simulink model "final_ekf_switch_test"  (R2024a)
settings: Solver=VariableStepAuto  StartTime=0.0  StopTime=10.0  RelTol=1e-3
undefined symbols (not defined in the file): DiscIntNeverNeededParam, g_val, Ki, Kx, m_val, r_pos
libraries: sharedTrackingLibrary x1
settings Model: Creator=yufon  LastModifiedBy=yufon

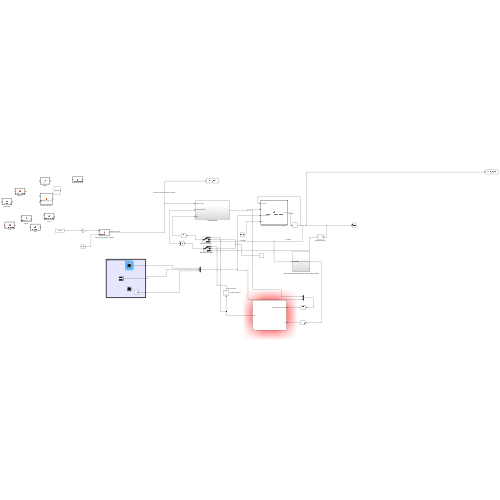
[thumbnail: Simulink's stored preview of the top-level diagram]
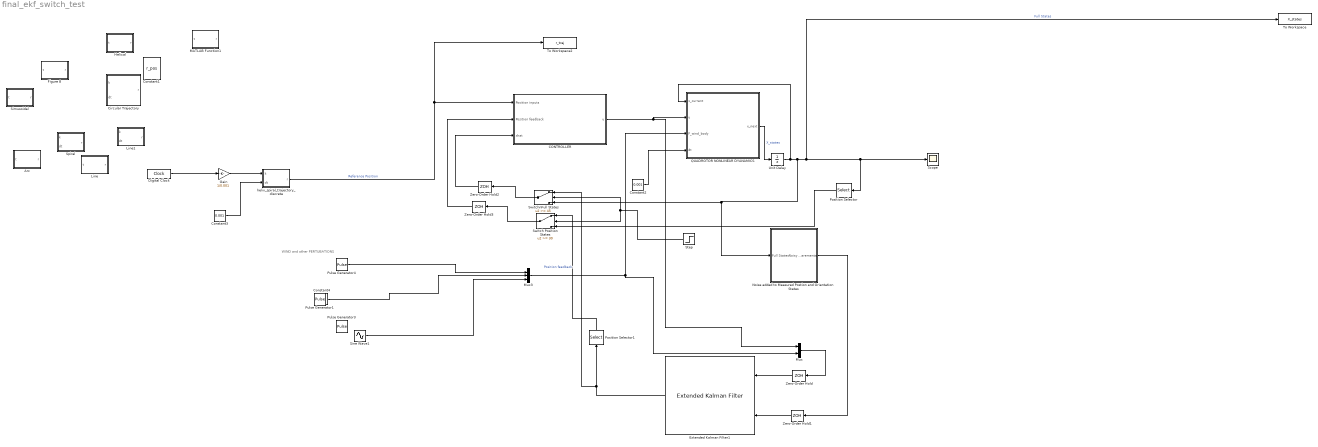
== system final_ekf_switch_test ==
  note: WIND and other PERTUBATIONS
  Arc : MATLAB Function  TreatAsAtomicUnit=on
  CONTROLLER : Subsystem
  Circular Trajectory : MATLAB Function  TreatAsAtomicUnit=on
  Constant1 : Constant  Value=r_pos  VectorParams1D=off
  Constant2 : Constant  Value=0.001
  Constant3 : Constant  Value=0.001
  Constant4 : Constant  Value=0
  Digital Clock : DigitalClock  SampleTime=0.01
  Extended Kalman Filter1 : sharedTrackingLibrary/Extended Kalman Filter  StateTransitionFcn=myStateTransitionFcn  HasStateTransitionJacobianFcn=off  HasAdditiveProcessNoise=Additive  ProcessNoise=Q  HasTimeVaryingProcessNoise=off  HasStateTransitionFcnExtraArgument=1  InitialState=EKF_x0  InitialStateCovariance=P0  MeasurementFcn1=myMeasurementFcn  HasMeasurementJacobianFcn1=off  HasMeasurementEnablePort1=off  HasAdditiveMeasurementNoise1=Additive  MeasurementNoise1=R  HasTimeVaryingMeasurementNoise1=off  HasMeasurementFcnExtraArgument1=0  HasMeasurementWrapping1=off  MeasurementFcn2=myMeasurementFcn  HasMeasurementJacobianFcn2=off  HasMeasurementEnablePort2=off  HasAdditiveMeasurementNoise2=Additive  MeasurementNoise2=1  HasTimeVaryingMeasurementNoise2=off  HasMeasurementFcnExtraArgument2=0  HasMeasurementWrapping2=off  MeasurementFcn3=myMeasurementFcn  HasMeasurementJacobianFcn3=off  HasMeasurementEnablePort3=off  HasAdditiveMeasurementNoise3=Additive  MeasurementNoise3=1  HasTimeVaryingMeasurementNoise3=off  HasMeasurementFcnExtraArgument3=0  HasMeasurementWrapping3=off  MeasurementFcn4=myMeasurementFcn  HasMeasurementJacobianFcn4=off  HasMeasurementEnablePort4=off  HasAdditiveMeasurementNoise4=Additive  MeasurementNoise4=1  HasTimeVaryingMeasurementNoise4=off  HasMeasurementFcnExtraArgument4=0  HasMeasurementWrapping4=off  MeasurementFcn5=myMeasurementFcn  HasMeasurementJacobianFcn5=off  HasMeasurementEnablePort5=off  HasAdditiveMeasurementNoise5=Additive  MeasurementNoise5=1  HasTimeVaryingMeasurementNoise5=off  HasMeasurementFcnExtraArgument5=0  HasMeasurementWrapping5=off  EnableMultirate=off  StateTransitionFcnSampleTime=1  MeasurementFcn1SampleTime=1  MeasurementFcn2SampleTime=1  MeasurementFcn3SampleTime=1  MeasurementFcn4SampleTime=1  MeasurementFcn5SampleTime=1  UseCurrentEstimator=on  OutputStateCovariance=off  DataType=double  SampleTime=0.001  NumberOfMeasurements=1
  Figure 8 : MATLAB Function  TreatAsAtomicUnit=on
  Gain : Gain  Gain=1/0.001
  Helical : MATLAB Function  TreatAsAtomicUnit=on
  Line : MATLAB Function  TreatAsAtomicUnit=on
  Line1 : MATLAB Function  TreatAsAtomicUnit=on
  MATLAB Function1 : MATLAB Function  TreatAsAtomicUnit=on
  Mux : Mux  Inputs=2
  Mux3 : Mux  Inputs=3
  Noise added to Measured Postion and Orientation States : Subsystem
  Position Selector : Selector  InputPortWidth=12  IndexOptions=Index vector (dialog)  Indices=[1 2 3]  OutputSizes=1
  Position Selector1 : Selector  InputPortWidth=12  IndexOptions=Index vector (dialog)  Indices=[1 2 3]  OutputSizes=1
  Pulse Generator1 : DiscretePulseGenerator  Amplitude=10  Period=10  PulseWidth=5  PhaseDelay=20  SampleTime=10
  Pulse Generator3 : DiscretePulseGenerator  PulseType=Time based  Amplitude=3  Period=5  PhaseDelay=100
  Pulse Generator4 : DiscretePulseGenerator  PulseType=Time based  Amplitude=3  Period=10  PulseWidth=5  PhaseDelay=50
  QUADROTOR NONLINEAR DYANAMICS : MATLAB Function  TreatAsAtomicUnit=on
  Scope : Scope
  Simusoidal : MATLAB Function  TreatAsAtomicUnit=on
  Sine Wave1 : Sin  Amplitude=5  Frequency=0.5  SampleTime=0
  Spiral : MATLAB Function  TreatAsAtomicUnit=on
  Step : Step  Time=45  After=30  SampleTime=0.001
  Switch Position States : Switch  Threshold=30  SaturateOnIntegerOverflow=off  InputSameDT=off
  SwitchnFull States : Switch  Threshold=45  SaturateOnIntegerOverflow=off  InputSameDT=off
  To Workspace : ToWorkspace  VariableName=X_states  SampleTime=-1
  To Workspace2 : ToWorkspace  VariableName=r_traj  SaveFormat=Timeseries  SampleTime=-1
  Unit Delay : UnitDelay  SampleTime=0.001  HasFrameUpgradeWarning=on
  Zero-Order Hold{,1..3} (4 alike) : ZeroOrderHold  SampleTime=0.001
  helix_spiral_trajectory_discrete : MATLAB Function  TreatAsAtomicUnit=on
  wires:
  Unit Delay/1 -> SwitchnFull States/3, Noise added to Measured Postion and Orientation States/1(Full States), Position Selector/1, Scope/1, To Workspace/1, QUADROTOR NONLINEAR DYANAMICS/1(x_current)  "Full States"
  SwitchnFull States/1 -> Zero-Order Hold2/1
  Extended Kalman Filter1/1 -> SwitchnFull States/1, Position Selector1/1
  helix_spiral_trajectory_discrete/1(r) -> To Workspace2/1, CONTROLLER/1(Position inputs)  "Reference Position"
  Constant3/1 -> helix_spiral_trajectory_discrete/2(dt)
  Zero-Order Hold3/1 -> CONTROLLER/2(Position feedback)
  Constant2/1 -> QUADROTOR NONLINEAR DYANAMICS/4(dt)
  Digital Clock/1 -> Gain/1
  Mux3/1 -> Mux/2, QUADROTOR NONLINEAR DYANAMICS/3(F_wind_body)
  Zero-Order Hold1/1 -> Extended Kalman Filter1/2
  Zero-Order Hold2/1 -> CONTROLLER/3(xhat)
  Mux/1 -> Zero-Order Hold/1
  Step/1 -> SwitchnFull States/2, Switch Position States/2
  Gain/1 -> helix_spiral_trajectory_discrete/1(k)
  Sine Wave1/1 -> Mux3/3
  CONTROLLER/1(u) -> Mux/1, QUADROTOR NONLINEAR DYANAMICS/2(u)
  Zero-Order Hold/1 -> Extended Kalman Filter1/1
  Constant4/1 -> Mux3/2
  Pulse Generator4/1 -> Mux3/1
  Position Selector/1 -> Switch Position States/3
  Position Selector1/1 -> Switch Position States/1  "Position feedback"
  Switch Position States/1 -> Zero-Order Hold3/1
  QUADROTOR NONLINEAR DYANAMICS/1(x_next) -> Unit Delay/1  "X_states"
  Noise added to Measured Postion and Orientation States/1(Noisy Position and Orientation Mesuarements) -> Zero-Order Hold1/1

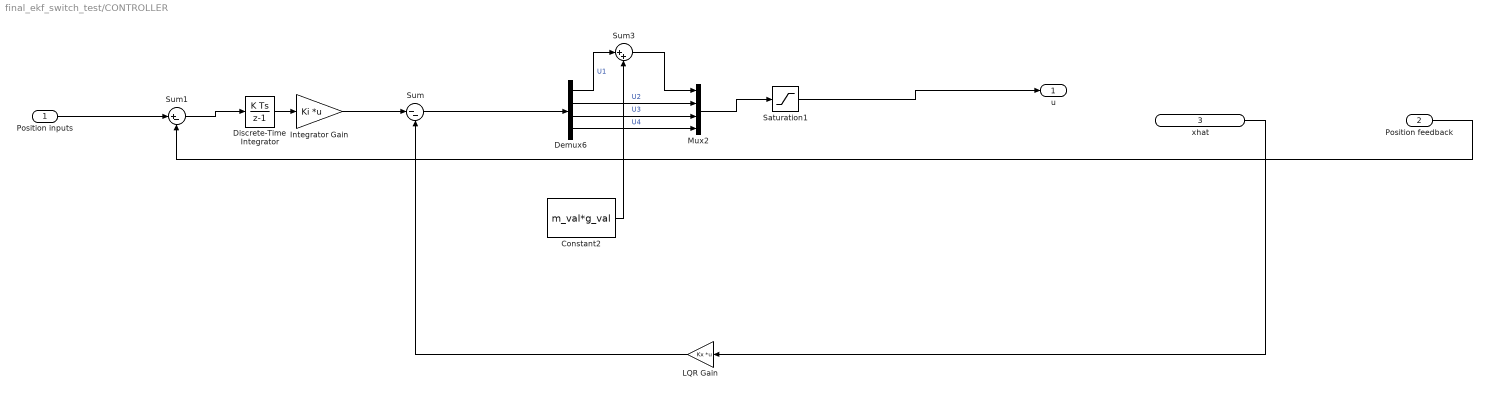
== system final_ekf_switch_test/CONTROLLER ==
  Position inputs : Inport
  Position feedback : Inport  Port=2
  xhat : Inport  Port=3
  Constant2 : Constant  Value=m_val*g_val
  Demux6 : Demux
  Discrete-Time Integrator : DiscreteIntegrator  SampleTime=0.001  ICPrevOutput=DiscIntNeverNeededParam  ICPrevScaledInput=DiscIntNeverNeededParam
  Integrator Gain : Gain  Gain=Ki  Multiplication=Matrix(K*u)
  LQR Gain : Gain  Gain=Kx  Multiplication=Matrix(K*u)
  Mux2 : Mux
  Saturation1 : Saturate  UpperLimit=[40; 0.15; 0.1;0.1]  LowerLimit=[0; -0.15; -0.10; -0.10]
  Sum : Sum  Inputs=|--
  Sum1 : Sum  Inputs=|+-
  Sum3 : Sum  Inputs=|++
  u : Outport
  wires:
  Constant2/1 -> Sum3/2
  LQR Gain/1 -> Sum/2
  Saturation1/1 -> u/1
  Demux6/4 -> Mux2/4  "U4"
  Mux2/1 -> Saturation1/1
  Demux6/2 -> Mux2/2  "U2"
  Discrete-Time Integrator/1 -> Integrator Gain/1
  Demux6/1 -> Sum3/1  "U1"
  Position feedback/1 -> Sum1/2
  Demux6/3 -> Mux2/3  "U3"
  Sum/1 -> Demux6/1
  Sum1/1 -> Discrete-Time Integrator/1
  Sum3/1 -> Mux2/1
  Integrator Gain/1 -> Sum/1
  Position inputs/1 -> Sum1/1
  xhat/1 -> LQR Gain/1

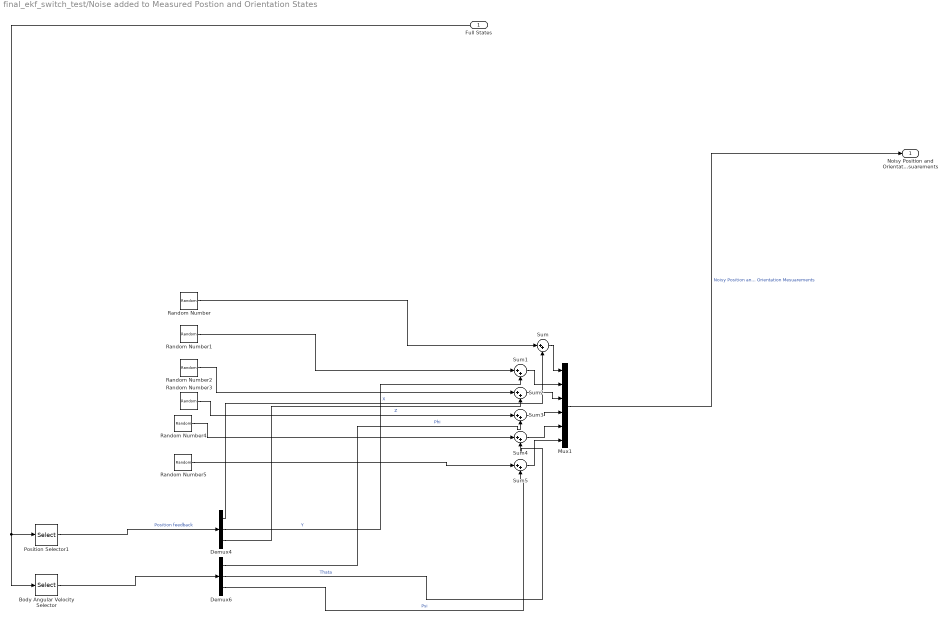
== system final_ekf_switch_test/Noise added to Measured Postion and Orientation States ==
  Full States : Inport
  Body Angular Velocity Selector : Selector  InputPortWidth=12  IndexOptions=Index vector (dialog)  Indices=[10 11 12]  OutputSizes=1
  Demux4 : Demux  Outputs=3
  Demux6 : Demux  Outputs=3
  Mux1 : Mux  Inputs=6
  Position Selector1 : Selector  InputPortWidth=12  IndexOptions=Index vector (dialog)  Indices=[1 2 3]  OutputSizes=1
  Random Number : RandomNumber  Variance=0.05*0.05  SampleTime=0.1
  Random Number1 : RandomNumber  Variance=0.05*0.05  SampleTime=0.1
  Random Number2 : RandomNumber  Variance=0.05*0.05  SampleTime=0.1
  Random Number3 : RandomNumber  Mean=0.01*0.01  SampleTime=0.1
  Random Number4 : RandomNumber  Mean=0.01*0.01  SampleTime=0.1
  Random Number5 : RandomNumber  Mean=0.01*0.01  SampleTime=0.1
  Sum{,1..5} (6 alike) : Sum  Inputs=|++
  Noisy Position and Orientation Mesuarements : Outport
  wires:
  Random Number1/1 -> Sum1/1
  Sum5/1 -> Mux1/6
  Demux6/3 -> Sum5/2  "Psi"
  Random Number2/1 -> Sum2/1
  Demux4/1 -> Sum/2  "X"
  Random Number3/1 -> Sum3/1
  Sum3/1 -> Mux1/4
  Sum1/1 -> Mux1/2
  Sum/1 -> Mux1/1
  Sum4/1 -> Mux1/5
  Sum2/1 -> Mux1/3
  Mux1/1 -> Noisy Position and Orientation Mesuarements/1  "Noisy Position and Orientation Mesuarements"
  Demux6/2 -> Sum4/2  "Thata"
  Random Number/1 -> Sum/1
  Demux4/2 -> Sum1/2  "Y"
  Demux4/3 -> Sum2/2  "Z"
  Demux6/1 -> Sum3/2  "Phi"
  Full States/1 -> Body Angular Velocity Selector/1, Position Selector1/1
  Random Number5/1 -> Sum5/1
  Body Angular Velocity Selector/1 -> Demux6/1
  Position Selector1/1 -> Demux4/1  "Position feedback"
  Random Number4/1 -> Sum4/1

== matlab function final_ekf_switch_test/Circular Trajectory ==
  data: k input; r output; dt input

function r = trajectory_discrete(k, dt)
    % Parameters (you can also pass these in or make them tunable)
    R = 5;          % Radius of circle (meters)
    omega = 0.1;    % Angular frequency (rad/s)
    z0 = 10;        % Base altitude (meters)
    A = 2;          % Amplitude of vertical oscillation (meters)
    omega_z = 0.05; % Vertical oscillation frequency (rad/s)
    x_offset = 0;   % Starting at x=0
    y_offset = 0;   % Starting at y=0
    z_offset = 0;   % Starting at z=0
    
    % Convert discrete step k to time
    t = k * dt;
    
    % Reference trajectory components
    r_x = x_offset + R * cos(omega * t);
    r_y = y_offset + R * sin(omega * t);
    r_z = z_offset + z0 + 0 * sin(omega_z * t); % Set A = 0 for pure circle
    
    % Output as a 3x1 vector
    r = [r_x; r_y; r_z];
end

== matlab function final_ekf_switch_test/Line ==
  data: t input; r output
function r = linear_ref(t)
    % Define total time and start/end positions
    T_total = 50;  % duration of trajectory
    r_start = [0; 0; 0];
    r_end   = [5; 5; 5];

    % Clamp progress between 0 and 1
    progress = min(max(t / T_total, 0), 1);

    % Linear interpolation
    r = r_start + (r_end - r_start) * progress;
end

== matlab function final_ekf_switch_test/MATLAB Function1 ==
  data: t input; r output
function r = rectangular_trajectory(t)
    % Rectangular trajectory parameters
    x_length = 10;       % Rectangle length (x-direction) in meters
    y_width = 8;         % Rectangle width (y-direction) in meters
    z_height = 5;        % Z height in meters
    duration = 500;       % Total duration in seconds
    
    % Add initial offset to match quadcopter starting position
    x_offset = 0;        % Starting at x=0
    y_offset = 0;        % Starting at y=0
    z_offset = 0;        % Starting at z=0
    
    % Time progression (clamped between 0 and 1)
    progress = min(max(t / duration, 0), 1);
    
    % Define the four segments of the rectangle
    % Each segment takes 25% of the total time
    if progress < 0.25 
        % First segment: Moving along x-axis (0 to x_length)
        segment_progress = progress / 0.25;
        x_ref = x_offset + x_length * segment_progress;
        y_ref = y_offset;
        z_ref = z_offset + z_height * segment_progress;
    elseif progress < 0.5
        % Second segment: Moving along y-axis (0 to y_width)
        segment_progress = (progress - 0.25) / 0.25;
        x_ref = x_offset + x_length;
        y_ref = y_offset + y_width * segment_progress;
        z_ref = z_offset + z_height;
    elseif progress < 0.75
        % Third segment: Moving along x-axis (x_length to 0)
        segment_progress = (progress - 0.5) / 0.25;
        x_ref = x_offset + x_length * (1 - segment_progress);
        y_ref = y_offset + y_width;
        z_ref = z_offset + z_height;
    else
        % Fourth segment: Moving along y-axis (y_width to 0)
        segment_progress = (progress - 0.75) / 0.25;
        x_ref = x_offset;
        y_ref = y_offset + y_width * (1 - segment_progress);
        z_ref = z_offset + z_height;
    end
    
    r = [x_ref; y_ref; z_ref];
end

== matlab function final_ekf_switch_test/QUADROTOR NONLINEAR DYANAMICS ==
  data: x_current input size=[12 1]; u input size=[4 1]; x_next output size=[12 1]; F_wind_body input; dt input
function x_next = quadrotor_dynamics_discrete(x_current, u, F_wind_body, dt)
    % Get the state derivatives from your continuous-time model
    dx = quadrotor_dynamics(u, x_current, F_wind_body);
    
    % Apply Forward Euler discretization
    x_next = x_current + dt * dx;
end

== matlab function final_ekf_switch_test/Line1 ==
  data: k input; r output; dt input
function r = spiral_trajectory_discrete(k, dt)
    % Parameters for spiral trajectory
    R_start = 1;       % Starting radius (meters)
    R_end = 5;         % Final radius (meters)
    omega = 0.1;       % Angular frequency (rad/s)
    z0 = 10;           % Constant altitude (meters)
    spiral_duration = 60; % Time to reach final radius (seconds)
    x_offset = 0;      % Center x-coordinate
    y_offset = 0;      % Center y-coordinate
    z_offset = 0;      % Base z-coordinate
    
    % Convert discrete step k to time
    t = k * dt;
    
    % Calculate radius (linear increase)
    radius = R_start + (R_end - R_start) * min(t/spiral_duration, 1);
    
    % Reference trajectory components
    r_x = x_offset + radius * cos(omega * t);
    r_y = y_offset + radius * sin(omega * t);
    r_z = z_offset + z0;
    
    % Output as a 3x1 vector
    r = [r_x; r_y; r_z];
end

== matlab function final_ekf_switch_test/Arc ==
  data: t input; r output
function r = arc_trajectory(t)
    % Arc parameters
    R = 5;
    theta_start = 0;
    theta_end = pi/2;
    duration = 10;
    z_const = 5;
    
    % Add initial offset to match quadcopter starting position
    x_offset = 0;  % Starting at x=0
    y_offset = 0;  % Starting at y=0
    z_offset = 0;  % Starting at z=0
    
    % Time progression
    progress = min(max(t / duration, 0), 1);
    theta = theta_start + progress * (theta_end - theta_start);
    
    % Reference position with offset
    x_ref = x_offset + (R * cos(theta) - R * cos(theta_start)) * progress;
    y_ref = y_offset + (R * sin(theta) - R * sin(theta_start)) * progress;
    z_ref = z_offset + z_const * progress;
    
    r = [x_ref; y_ref; z_ref];
end

== matlab function final_ekf_switch_test/Simusoidal ==
  data: t input; r output
function r = sinusoidal_trajectory(t)
    % Sinusoidal trajectory with varying frequencies
    % Parameters
    x_amp = 5;           % X amplitude in meters
    y_amp = 3;           % Y amplitude in meters
    z_max = 5;           % Maximum z height in meters
    duration = 500;       % Total duration in seconds
    
    % Frequency parameters
    f_start = 0.1;       % Starting frequency in Hz
    f_end = 0.5;         % Ending frequency in Hz
    
    % Add initial offset to match quadcopter starting position
    x_offset = 0;        % Starting at x=0
    y_offset = 0;        % Starting at y=0
    z_offset = 0;        % Starting at z=0
    
    % Time progression (clamped between 0 and 1)
    progress = min(max(t / duration, 0), 1);
    
    % Varying frequency over time (linear interpolation)
    current_freq = f_start + progress * (f_end - f_start);
    
    % Phase shift to ensure y is 90 degrees out of phase with x
    phase_shift = pi/2;
    
    % Calculate positions
    x_ref = x_offset + x_amp * sin(2 * pi * current_freq * t);
    y_ref = y_offset + y_amp * sin(2 * pi * current_freq * t + phase_shift);
    z_ref = z_offset + z_max * progress;
    
    r = [x_ref; y_ref; z_ref];
end

== matlab function final_ekf_switch_test/Spiral ==
  data: k input; r output; dt input
function r = spiral_trajectory_discrete(k, dt)
    % Spiral Trajectory Generator (Discrete Version)
    
    % Parameters
    R = 5;           % Radius of spiral (constant)
    duration = 500;  % Total time for spiral traversal
    turns = 2;       % Number of full 2π turns
    height = 5;      % Total height climbed
    
    % Convert discrete step k to time
    t = k * dt;
    
    % Time normalization
    progress = min(max(t / duration, 0), 1);
    
    % Angle progresses from 0 to 2π * turns
    theta = progress * (2 * pi * turns);
    
    % Spiral path in x, y and ascending in z
    x_ref = R * cos(theta);
    y_ref = R * sin(theta);
    z_ref = height * progress;
    
    % Output reference position
    r = [x_ref; y_ref; z_ref];
end

== matlab function final_ekf_switch_test/Figure 8 ==
  data: t input; r output
function r = figure_eight_trajectory(t)
    % Parameters
    R = 5;               % Radius of the loops
    omega = 0.2;         % Angular speed [rad/s]
    duration = 500;       % Total time to complete one figure-eight
    z_const = 5;         % Constant height
    
    % Initial offset (optional)
    x_offset = 0;
    y_offset = 0;
    z_offset = 0;

    % Time progression
    progress = min(max(t / duration, 0), 1);
    theta = omega * t;

    % Figure-eight Lissajous shape
    x_ref = x_offset + R * sin(theta);
    y_ref = y_offset + R * sin(theta) .* cos(theta);
    z_ref = z_offset + z_const;

    r = [x_ref; y_ref; z_ref];
end

== matlab function final_ekf_switch_test/Helical ==
  data: t input; r output
function r = helical_trajectory(t)
    % Parameters
    R = 5;              % Radius in meters
    omega = 2 * pi / 20; % Angular speed (rad/s) for smooth loops
    z_max = 10;         % Max height
    duration = 500;     % Total trajectory time in seconds

    % Time progress normalized
    progress = min(max(t / duration, 0), 1);
    theta = omega * t;

    % Reference position, offset to start at (0, 0, 0)
    x_ref = R * (cos(theta) - 1);   % cos(0) - 1 = 0
    y_ref = R * sin(theta);
    z_ref = z_max * progress;

    r = [x_ref; y_ref; z_ref];
end

== matlab function final_ekf_switch_test/helix_spiral_trajectory_discrete ==
  data: k input; r output; dt input
function r = helix_spiral_trajectory_discrete(k, dt)
    % Helix Spiral Trajectory Generator (Discrete Version)
    
    % Parameters
    R = 5;           % Radius of spiral (meters)
    duration = 500;   % Total time for spiral traversal (seconds)
    turns = 2;       % Number of full 2π turns
    height = 5;      % Total height to climb (meters)
    
    % Convert discrete step k to time
    t = k * dt;
    
    % Calculate progress (clamped between 0 and 1)
    progress = min(max(t / duration, 0), 1);
    
    % Calculate angle (increases with time)
    theta = progress * (2 * pi * turns);
    
    % Calculate position components
    x_ref = R * cos(theta);
    y_ref = R * sin(theta);
    z_ref = height * progress;  % Linear increase in height
    
    % Output reference position as a 3×1 vector
    r = [x_ref; y_ref; z_ref];
end
